simulink model "workshop6_DCMotor_deriv"  (R2026a)
settings: Solver=VariableStepAuto  StopTime=0.5
values from neighbouring files (symbols this model uses):
  C = kp + ki/s + (kd*s)/(1+s*Tf)    [workshop6_deriv_setupParams.m]    (also in workshop6_discretisedCtl_setupParams.m = kd*s/(Tf*s+1) + kp + ki/s)
  S_simple = (K/R)/(J*s+b+(K^2)/R)    [workshop6_deriv_setupParams.m]    (also in workshop6_discretisedCtl_setupParams.m)
libraries: simulink x2
settings Model: Creator=leoyi  LastModifiedBy=socks

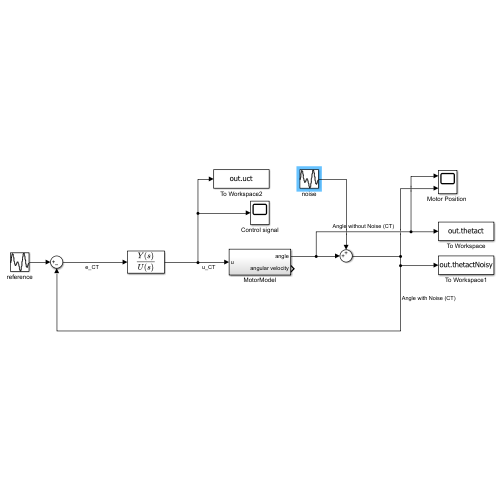
[thumbnail: Simulink's stored preview of the top-level diagram]
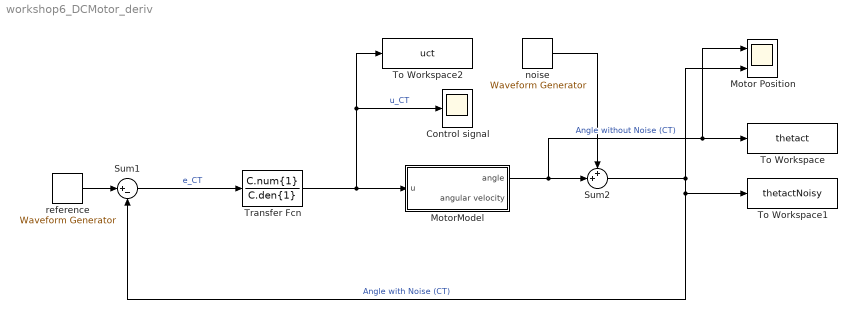
== system workshop6_DCMotor_deriv ==
  Control signal : Scope
      settings: ActiveDisplayYMinimum=-11.08461  ActiveDisplayYMaximum=24.56496  DataLoggingVariableName=ScopeData2
  "Motor Position " : Scope  NumInputPorts=2
      settings: ActiveDisplayYMinimum=-0.12365  ActiveDisplayYMaximum=1.11288
  MotorModel : Subsystem
  Sum1 : Sum  Inputs=|+-
  Sum2 : Sum  Inputs=++|
  To Workspace : ToWorkspace  VariableName=thetact  SaveFormat=Timeseries  SampleTime=-1
  To Workspace1 : ToWorkspace  VariableName=thetactNoisy  SaveFormat=Timeseries  SampleTime=-1
  To Workspace2 : ToWorkspace  VariableName=uct  SaveFormat=Timeseries  SampleTime=-1
  Transfer Fcn : TransferFcn  Numerator=C.num{1}  Denominator=C.den{1}
  noise : simulink/Sources/Waveform Generator  OutMin=[]  OutMax=[]  OutDataTypeStr=double  SelectedSignal=2  Signals=gaussian('Mean',0,'Variance',0.0025)#0  BlockNames=MultiportSwitch_ca9fcf45f272486#MultiportSwitch_cd333301a39a4eb  SampleTime=0.001
  reference : simulink/Sources/Waveform Generator  OutMin=[]  OutMax=[]  OutDataTypeStr=double  SelectedSignal=2  Signals=1#square('Amplitude',1,'Frequency',2*pi/0.25,'Phase',0,'DutyCycle',50)  BlockNames=MultiportSwitch_5740d72aaa054f2#MultiportSwitch_ba4dfc40e38844e  SampleTime=0.001
  wires:
  reference/1 -> Sum1/1
  Sum1/1 -> Transfer Fcn/1  "e_CT"
  noise/1 -> Sum2/1
  MotorModel/1(angle) -> "Motor Position "/1, To Workspace/1, Sum2/2  "Angle without Noise (CT)"
  Sum2/1 -> "Motor Position "/2, To Workspace1/1, Sum1/2  "Angle with Noise (CT)"
  Transfer Fcn/1 -> To Workspace2/1, Control signal/1, MotorModel/1(u)  "u_CT"

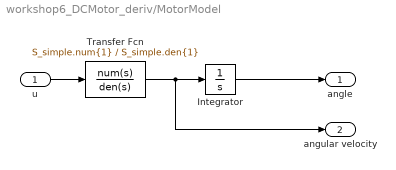
== system workshop6_DCMotor_deriv/MotorModel ==
  u : Inport
  Integrator : Integrator
  Transfer Fcn : TransferFcn  Numerator=S_simple.num{1}  Denominator=S_simple.den{1}
  angle : Outport
  angular velocity : Outport  Port=2
  wires:
  u/1 -> Transfer Fcn/1
  Transfer Fcn/1 -> angular velocity/1, Integrator/1
  Integrator/1 -> angle/1
